simulink model "avlAerodynamics6D_th"  (R2022a)
settings: Solver=VariableStepAuto  StartTime=0.0  StopTime=0  RelTol=1e-3
values from neighbouring files (symbols this model uses):
  ailDefl_deg = 0    [avlAerodynamics6D_ts.m]
  dynPress = 1    [avlAerodynamics6D_ts.m]
  elevDefl_deg = 0    [avlAerodynamics6D_ts.m]
  flpDefl_deg = 0    [avlAerodynamics6D_ts.m]
  rudDefl_deg = 0    [avlAerodynamics6D_ts.m]
  uAppBdy = [5 0 1]    [avlAerodynamics6D_ts.m]
libraries: avlAerodynamics6D x1
settings Model: Creator=mcobb  LastModifiedBy=lhill8
settings SolverCC: AlgebraicLoopSolver=TrustRegion
settings DebuggingCC: UnconnectedInputMsg=warning  UnconnectedOutputMsg=warning  UnconnectedLineMsg=warning  SFMachineParentedDataDiag=warning  ArithmeticOperatorsInVariantConditions=warning
settings SFSimCC: CustomCodeUndefinedFunction=UseInterfaceOnly

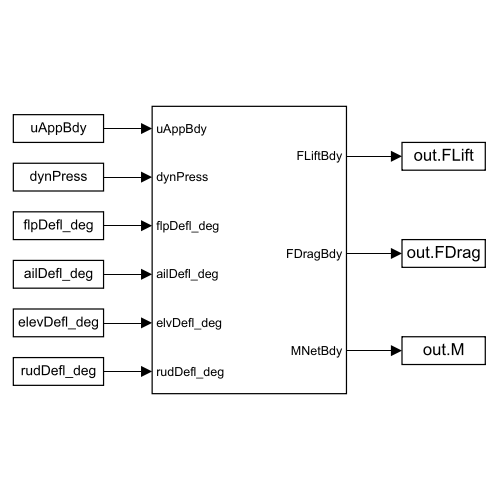
[thumbnail: Simulink's stored preview of the top-level diagram]
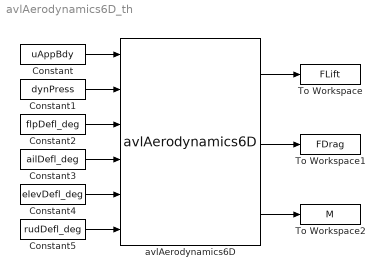
== system avlAerodynamics6D_th ==
  Constant : Constant  Value=uAppBdy
  Constant1 : Constant  Value=dynPress
  Constant2 : Constant  Value=flpDefl_deg
  Constant3 : Constant  Value=ailDefl_deg
  Constant4 : Constant  Value=elevDefl_deg
  Constant5 : Constant  Value=rudDefl_deg
  To Workspace : ToWorkspace  VariableName=FLift  SaveFormat=Timeseries  SampleTime=-1
  To Workspace1 : ToWorkspace  VariableName=FDrag  SaveFormat=Timeseries  SampleTime=-1
  To Workspace2 : ToWorkspace  VariableName=M  SaveFormat=Timeseries  SampleTime=-1
  avlAerodynamics6D : avlAerodynamics6D/avlAerodynamics6D  CLTable=CLtotTbl  CDTable=CLtotTbl  CMxTable=CLtotTbl  CMyTable=CLtotTbl  CMzTable=CLtotTbl  SRef=0  BRef=0  CRef=0
  wires:
  Constant/1 -> avlAerodynamics6D/1
  Constant4/1 -> avlAerodynamics6D/5
  Constant3/1 -> avlAerodynamics6D/4
  Constant2/1 -> avlAerodynamics6D/3
  Constant1/1 -> avlAerodynamics6D/2
  avlAerodynamics6D/3 -> To Workspace2/1
  avlAerodynamics6D/2 -> To Workspace1/1
  avlAerodynamics6D/1 -> To Workspace/1
  Constant5/1 -> avlAerodynamics6D/6
